simulink model "untitled"  (Simulink 7.8)
settings: Solver=ode45  StartTime=0.0  StopTime=10.0  RelTol=1e-3
undefined symbols (not defined in the file or in its folder): Bar1_length, Load_torque, Motor_speed, Stall_torque
libraries: mblibv1 x8, fl_lib x4, simulink x2, mech_friction x1, nesl_utility x1
settings Model: Creator=ftian  LastModifiedBy=ftian

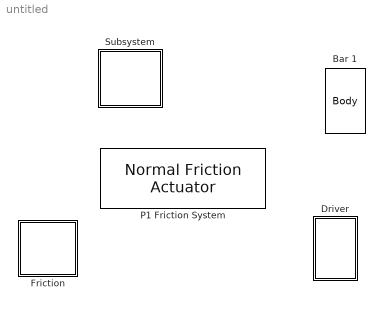
== system untitled ==
  Bar 1 : mblibv1/Bodies/Body  LConnTagsString=CS1  RConnTagsString=CS2  UpdateFromCAD=off  DialogClass=MechanicalBodyBlock  Mass=1  MassUnits=g  InertiaUnits=g*cm^2  Inertia=[0.04 0 0;0 0.04 0;0 0 0.055]  Shape=Cylinder  ShapeDims=[1 1]  ShapeUnits=m  ShapeUse=false  Density=1  DensityUnits=kg/m^3  DensityUse=false  GraphicsMode=MACHINE_DEFAULT  BodyColorSelMode=COLORPALETTE  BodyColor=[0.87059 0.4902 0]  AttachedToCS=CG  CG=Left$CG$[0 0 Bar1_length/2]$CS1$CS1$mm$[0 0 0]$Euler X-Y-Z$deg$WORLD$false$none  WorkingFrames=Left$CS1$[0 0 0]$Adjoining$Adjoining$mm$[0 0 0]$Euler X-Y-Z$deg$WORLD$true$none#Right$CS2$[0 0 Bar1_length]$CS1$CS1$mm$[0 0 0]$Euler X-Y-Z$deg$WORLD$true$none  CGPos=[0 0 Bar1_length/2]  CGRot=[0 0 0]  CS0Pos=[]  CS0Rot=[]  CS1Pos=[0 0 0]  CS1Rot=[0 0 0]  CS2Pos=[0 0 Bar1_length]  CS2Rot=[0 0 0]  CS3Pos=[]  CS3Rot=[]  CS4Pos=[]  CS4Rot=[]  CS5Pos=[]  CS5Rot=[]  CS6Pos=[]  CS6Rot=[]  CS7Pos=[]  CS7Rot=[]  CS8Pos=[]  CS8Rot=[]  CS9Pos=[]  CS9Rot=[]  CS10Pos=[]  CS10Rot=[]  CS11Pos=[]  CS11Rot=[]  CS12Pos=[]  CS12Rot=[]  CS13Pos=[]  CS13Rot=[]  CS14Pos=[]  CS14Rot=[]  CS15Pos=[]  CS15Rot=[]  CS16Pos=[]  CS16Rot=[]  CS17Pos=[]  CS17Rot=[]  CS18Pos=[]  CS18Rot=[]  CS19Pos=[]  CS19Rot=[]  CS20Pos=[]  CS20Rot=[]
  Driver : Subsystem
  Friction : Subsystem
  P1 Friction System : mech_friction/Normal Friction Actuator  Ckinetic=0.1  staticFF=1.65  Csforward=0.055  Csreverse=0.055  sExtActuation=off  sForces=on  primitive=P1
  Subsystem : Subsystem

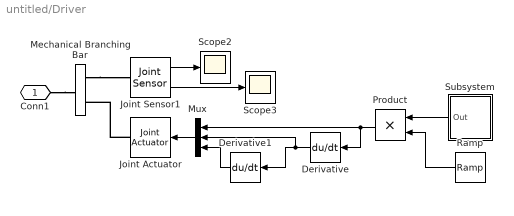
== system untitled/Driver ==
  Derivative : Derivative
  Derivative1 : Derivative
  Joint Actuator : mblibv1/Sensors &  Actuators/Joint Actuator  UpdateFromCAD=off  PhysicalDomain=Mechanical  PortType=blob  ActuationStyle=Motion  AngleUnits=rev  ArcVelocityUnits=rpm  ArcAccelerationUnits=deg/s^2  CoordPositionUnits=m  VelocityUnits=m/s  AccelerationUnits=m/s^2  ForceUnits=N  TorqueUnits=mN*m  ActiveIO=off  Width=3  DialogClass=MechanicalActuatorBlock  Primitive=R1  ReferenceFrame=Absolute (World)
  Joint Sensor1 : mblibv1/Sensors &  Actuators/Joint Sensor  UpdateFromCAD=off  PhysicalDomain=Mechanical  PortType=blob  Muxed=off  Pose=off  Angle=on  AngleUnits=deg  ArcVelocity=on  ArcVelocityUnits=rpm  ArcAcceleration=off  ArcAccelerationUnits=deg/s^2  CoordPosition=on  CoordPositionUnits=m  Velocity=off  VelocityUnits=m/s  Acceleration=off  AccelerationUnits=m/s^2  Quaternion=on  QuaternionDT=off  QuaternionDDT=off  QuaternionUnits=off  OutputVector=[1]  ActiveIO=off  Width=2  DialogClass=MechanicalSensorBlock  Primitive=R1  Force=off  ForceUnits=N  Torque=off  TorqueUnits=N*m  ReferenceFrame=Absolute (World)  ReactionSensedSide=Base  ReactionReferenceFrame=Absolute (World)  ReactionForce=off  ReactionForceUnits=N  ReactionMoment=off  ReactionMomentUnits=N*m
  Mechanical Branching Bar : mblibv1/Utilities/Mechanical Branching Bar  LConnTagsString=_newl0  RConnTagsString=__newr0|SA2  UpdateFromCAD=off  DialogClass=MechanicalBranchingBarBlock  NumSAPorts=2
  Mux : Mux  Inputs=3
  Product : Product  RndMeth=Zero
  Ramp : simulink/Sources/Ramp  slope=1  start=1  X0=0
  Scope2 : Scope
      settings: TimeRange=1  YMin=-4  YMax=3.5
  Scope3 : Scope
      settings: TimeRange=1  YMin=-4  YMax=3.5  SaveName=ScopeData2
  Subsystem : Subsystem
  Conn1 : PMIOPort  Port=1  Side=Left
  wires:
  Joint Sensor1/1 -> Scope2/1
  Derivative/1 -> Mux/2, Derivative1/1
  Derivative1/1 -> Mux/3
  Joint Sensor1/2 -> Scope3/1
  Mux/1 -> Joint Actuator/1
  Product/1 -> Mux/1, Derivative/1
  Subsystem/1(Out) -> Product/1
  Ramp/1 -> Product/2
  connections:
  Joint Actuator/RConn1 -- Mechanical Branching Bar/RConn2
  Mechanical Branching Bar/RConn1 -- Joint Sensor1/LConn1
  Conn1/RConn1 -- Mechanical Branching Bar/LConn1

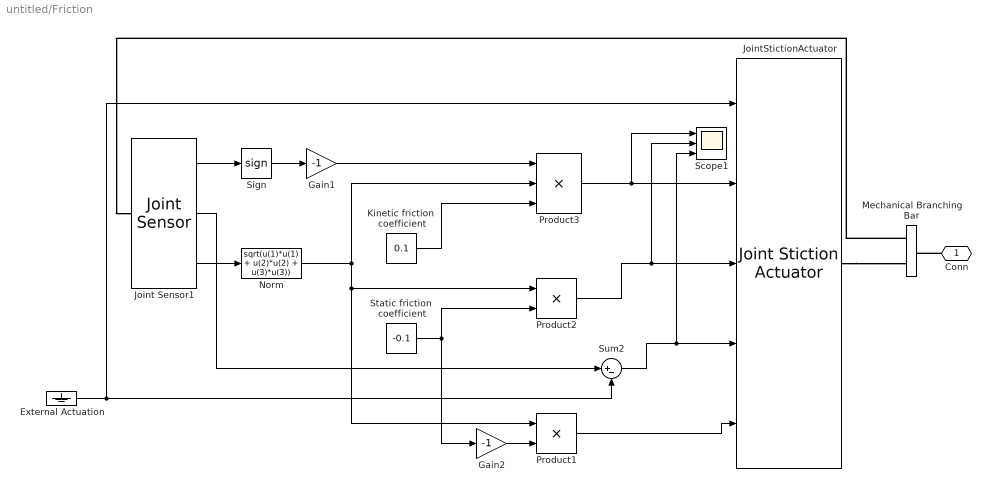
== system untitled/Friction ==
  External Actuation : Ground
  Gain1 : Gain  Gain=-1  SaturateOnIntegerOverflow=on  OutDataTypeStr=Inherit: Same as input  ParamDataTypeStr=Inherit: Same as input
  Gain2 : Gain  Gain=-1  SaturateOnIntegerOverflow=on  OutDataTypeStr=Inherit: Same as input  ParamDataTypeStr=Inherit: Same as input
  Joint Sensor1 : mblibv1/Sensors &  Actuators/Joint Sensor  UpdateFromCAD=off  PhysicalDomain=Mechanical  PortType=blob  Muxed=off  Pose=off  Angle=off  AngleUnits=deg  ArcVelocity=on  ArcVelocityUnits=deg/s  ArcAcceleration=off  ArcAccelerationUnits=deg/s^2  CoordPosition=on  CoordPositionUnits=m  Velocity=off  VelocityUnits=m/s  Acceleration=off  AccelerationUnits=m/s^2  Quaternion=on  QuaternionDT=off  QuaternionDDT=off  QuaternionUnits=off  OutputVector=[1]  ActiveIO=off  Width=5  DialogClass=MechanicalSensorBlock  Primitive=R1  Force=off  ForceUnits=N  Torque=on  TorqueUnits=mN*m  ReferenceFrame=Absolute (World)  ReactionSensedSide=Follower  ReactionReferenceFrame=Local (Body CS)  ReactionForce=on  ReactionForceUnits=mN  ReactionMoment=off  ReactionMomentUnits=mN*m
  JointStictionActuator : mblibv1/Sensors &  Actuators/Joint Stiction Actuator  UpdateFromCAD=off  PhysicalDomain=Mechanical  PortType=blob  ActuationStyle=Force  AngleUnits=deg  ArcVelocityUnits=deg/s  ArcAccelerationUnits=deg/s^2  CoordPositionUnits=m  VelocityUnits=m/s  AccelerationUnits=m/s^2  ForceUnits=N  TorqueUnits=N-m  ActiveIO=off  Width=5  DialogClass=EventActuatorBlock  Primitive=R1  FrictionalForceUnits=N  ExternalForceUnits=N  FrictionalTorqueUnits=mN*m  ExternalTorqueUnits=mN*m  LockingTolerance=1e-2
      link override MSB_SIGNAL_BLOCK: GotoTag=sim_mech_tag6f78254795838dc  TagVisibility=global
  Kinetic friction  coefficient : Constant  Value=0.1
  Mechanical Branching Bar : mblibv1/Utilities/Mechanical Branching Bar  LConnTagsString=_newl0  RConnTagsString=__newr0|SA2  UpdateFromCAD=off  DialogClass=MechanicalBranchingBarBlock  NumSAPorts=2
  Norm : Fcn  Expr=sqrt(u(1)*u(1) + u(2)*u(2) + u(3)*u(3))
  Product1 : Product  SaturateOnIntegerOverflow=on  InputSameDT=on  OutDataTypeStr=Inherit: Same as first input
  Product2 : Product  SaturateOnIntegerOverflow=on  InputSameDT=on  OutDataTypeStr=Inherit: Same as first input
  Product3 : Product  Inputs=3  SaturateOnIntegerOverflow=on  InputSameDT=on  OutDataTypeStr=Inherit: Same as first input
  Scope1 : Scope  NumInputPorts=3
      settings: TimeRange=1  YMin=-1~-66.6739~2  YMax=1~-66.6739~2
  Sign : Signum  ZeroCross=off
  "Static friction  coefficient " : Constant  Value=-0.1
  Sum2 : Sum  Inputs=|+-  SaturateOnIntegerOverflow=on  InputSameDT=on  OutDataTypeStr=Inherit: Same as first input
  Conn : PMIOPort  Port=1  Side=Left
  wires:
  Joint Sensor1/1 -> Sign/1
  Sign/1 -> Gain1/1
  Gain1/1 -> Product3/1
  Joint Sensor1/3 -> Norm/1
  Norm/1 -> Product3/2, Product2/1, Product1/1
  Kinetic friction  coefficient/1 -> Product3/3
  "Static friction  coefficient "/1 -> Product2/2, Gain2/1
  Joint Sensor1/2 -> Sum2/1
  External Actuation/1 -> Sum2/2, JointStictionActuator/1
  Gain2/1 -> Product1/2
  Product3/1 -> JointStictionActuator/2, Scope1/1
  Product2/1 -> JointStictionActuator/3, Scope1/2
  Sum2/1 -> JointStictionActuator/4, Scope1/3
  Product1/1 -> JointStictionActuator/5
  connections:
  Conn/RConn1 -- Mechanical Branching Bar/LConn1
  JointStictionActuator/RConn1 -- Mechanical Branching Bar/RConn2
  Mechanical Branching Bar/RConn1 -- Joint Sensor1/LConn1

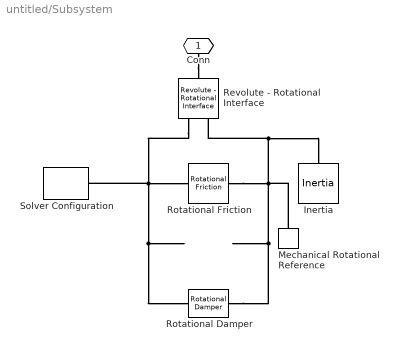
== system untitled/Subsystem ==
  Inertia : fl_lib/Mechanical/Rotational Elements/Inertia  inertia=1 g*cm^2  initial_velocity=0 rad/s  t_Log=off  LocalVarNames=|t  LocalVarDescs=|t  LocalVarLogging=0
  Mechanical Rotational Reference : fl_lib/Mechanical/Rotational Elements/Mechanical Rotational Reference  t_Log=off  LocalVarNames=|t  LocalVarDescs=|t  LocalVarLogging=0
  Revolute - Rotational Interface : mblibv1/Interface  Elements/Revolute - Rotational Interface  UpdateFromCAD=off  DialogClass=RevoluteRotationalInterface  Primitive=R1
  Rotational Damper : fl_lib/Mechanical/Rotational Elements/Rotational Damper  D=0.001 N*m/(rad/s)  t_Log=off  w_Log=off  LocalVarNames=|t|w  LocalVarDescs=|t|w  LocalVarLogging=[0 0]
  Rotational Friction : fl_lib/Mechanical/Rotational Elements/Rotational Friction  brkwy_trq=2 mN*m  Col_trq=1 mN*m  visc_coef=0.001 N*m/(rad/s)  trans_coef=10 s/rad  vel_thr=1e-4 rad/s  t_Log=off  w_Log=off  LocalVarNames=|t|w  LocalVarDescs=|t|w  LocalVarLogging=[0 0]
  Solver Configuration : nesl_utility/Solver Configuration  PhysicalDomain=network_engine_domain  LeftPortType=input  RightPortType=generic  SubClassName=solver  DoDC=off  ResidualTolerance=1e-9  UseLocalSolver=on  LocalSolverChoice=NE_BACKWARD_EULER_ADVANCER  LocalSolverSampleTime=.001  DoFixedCost=on  MaxNonlinIter=3  MaxModeIter=2  LinearAlgebra=Sparse  Accelerate=off  Profile=off  UseLocalSampling=off  DelaysMemoryBudget=1024
  Conn : PMIOPort  Port=1  Side=Right
  connections:
  Conn/RConn1 -- Revolute - Rotational Interface/RConn1
  Revolute - Rotational Interface/LConn1 -- Rotational Damper/LConn1 -- Rotational Friction/LConn1 -- Solver Configuration/RConn1
  Mechanical Rotational Reference/LConn1 -- Rotational Damper/RConn1 -- Rotational Friction/RConn1 -- Inertia/LConn1 -- Revolute - Rotational Interface/LConn2

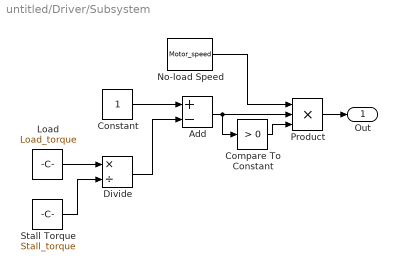
== system untitled/Driver/Subsystem ==
  Add : Sum  Inputs=+-
  Compare To Constant : simulink/Logic and Bit Operations/Compare To Constant  relop=>  const=0  OutDataTypeStr=uint8
  Constant : Constant
  Divide : Product  Inputs=*/
  Load : Constant  Value=Load_torque
  No-load Speed : Constant  Value=Motor_speed
  Product : Product  Inputs=3  RndMeth=Zero
  Stall Torque : Constant  Value=Stall_torque
  Out : Outport
  wires:
  Constant/1 -> Add/1
  Load/1 -> Divide/1
  Stall Torque/1 -> Divide/2
  Divide/1 -> Add/2
  Add/1 -> Product/2, Compare To Constant/1
  Product/1 -> Out/1
  Compare To Constant/1 -> Product/3
  No-load Speed/1 -> Product/1
